simulink model "rocky_motor_disturb"  (R2021b)
settings: Solver=VariableStepAuto  StartTime=0.0  StopTime=2  RelTol=1e-3
model workspace (MAT data in the model file):
  m = 1000
values from neighbouring files (symbols this model uses):
  g = 9.81    [Rocky_closed_loop_poles.m]    (also in rocky_constants.m)
  ki = real(1.241009049348965e+05)    [rocky_constants.m]
  kmotor = .0025    (= 0.0025)    [rocky_constants.m]
  kp = real(1.240922125348965e+05)    [rocky_constants.m]
  l = 22*2.54/100    (= 0.5588)    [Rocky_closed_loop_poles.m]    (also in rocky_constants.m)
  tau = 0.0958    [rocky_constants.m]
settings Model: Creator=clee1  LastModifiedBy=spoka
settings SolverCC: AlgebraicLoopSolver=TrustRegion
settings DebuggingCC: SFMachineParentedDataDiag=warning

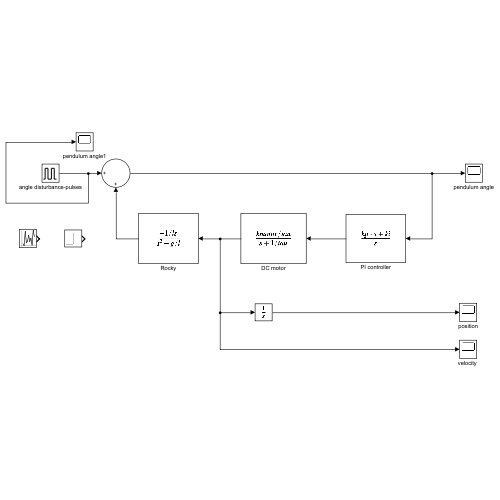
[thumbnail: Simulink's stored preview of the top-level diagram]
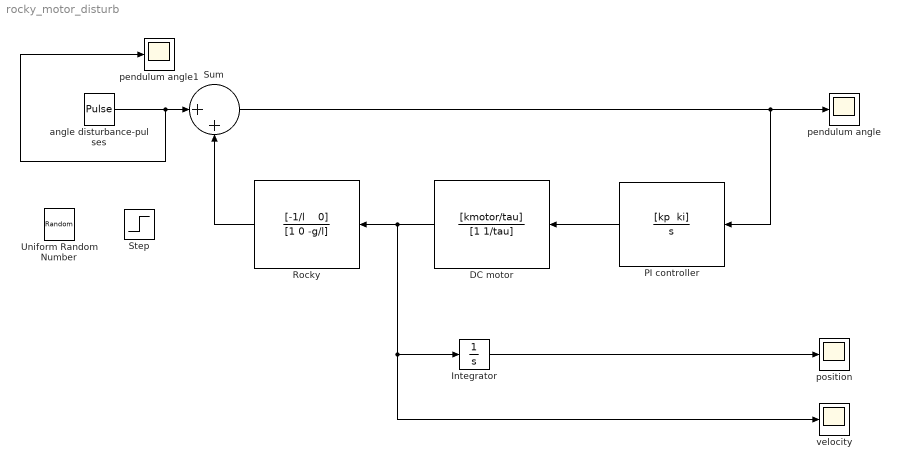
== system rocky_motor_disturb ==
  DC motor : TransferFcn  Numerator=[kmotor/tau]  Denominator=[1 1/tau]
  Integrator : Integrator
  PI controller : TransferFcn  Numerator="[kp  ki]"  Denominator=[1 0 ]
  Rocky : TransferFcn  Numerator="[-1/l    0]"  Denominator=[1 0 -g/l]
  Step : Step  After=.1  SampleTime=0
  Sum : Sum  Inputs=|++
  Uniform Random Number : UniformRandomNumber  SampleTime=20
  angle disturbance-pulses : DiscretePulseGenerator  PulseType=Time based  Amplitude=.1  Period=10  PulseWidth=.1  PhaseDelay=.5
  pendulum angle : Scope
  pendulum angle1 : Scope
  position : Scope
  "velocity " : Scope
  wires:
  Rocky/1 -> Sum/2
  Sum/1 -> PI controller/1, pendulum angle/1
  DC motor/1 -> "velocity "/1, Integrator/1, Rocky/1
  PI controller/1 -> DC motor/1
  Integrator/1 -> position/1
  angle disturbance-pulses/1 -> pendulum angle1/1, Sum/1
